simulink model "Juarez_22210417"  (R2023a)
settings: Solver=ode15s  StartTime=0.0  StopTime=30  MaxStep=1e-3  RelTol=1e-3
libraries: slpidlib x1
settings Model: Creator=edang  LastModifiedBy=edang
settings DataIOCC: ReturnWorkspaceOutputs=off  TimeSaveName=t
settings DebuggingCC: AlgebraicLoopMsg=none  ArtificialAlgebraicLoopMsg=none  MaxConsecutiveZCsMsg=none  ModelReferenceExtraNoncontSigs=none  OperatingPointInterfaceChecksumMismatchMsg=none

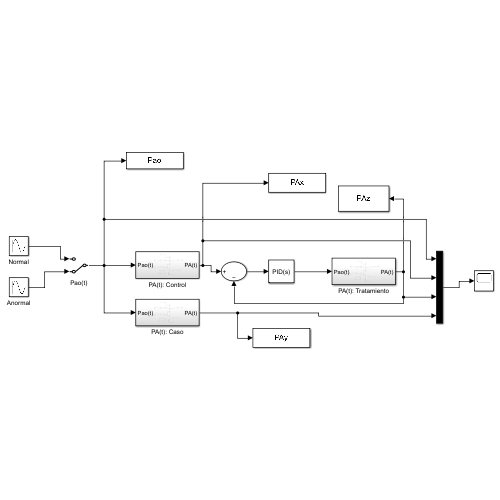
[thumbnail: Simulink's stored preview of the top-level diagram]
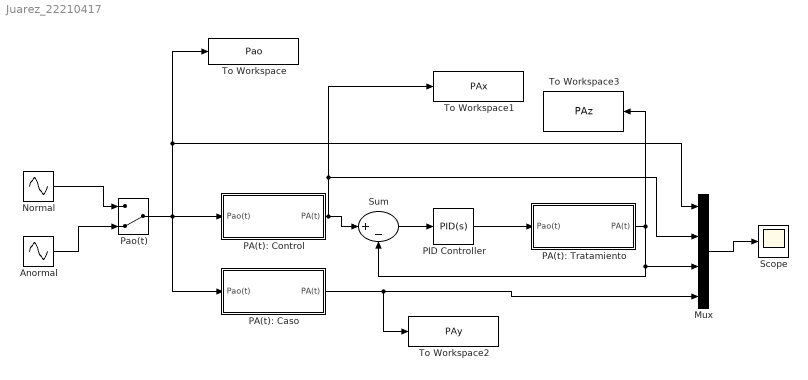
== system Juarez_22210417 ==
  Anormal : Sin  Amplitude=1.5  Frequency=pi/2  SampleTime=0
  Mux : Mux
  Normal : Sin  Amplitude=2.5  Frequency=pi  SampleTime=0
  PA(t): Caso : Subsystem
  PA(t): Control : Subsystem
  PA(t): Tratamiento : Subsystem
  PID Controller : slpidlib/PID Controller  Controller=PID  Form=Parallel  TimeDomain=Continuous-time  UseExternalTs=off  SampleTime=-1  IntegratorMethod=Forward Euler  FilterMethod=Forward Euler  ControllerParametersSource=internal  P=1874.1952  I=62315.7871  UseKiTs=off  D=8.8936  N=202877.133267727  UseFilter=on  TunerSelectOption=Transfer Function Based (PID Tuner App)  InitialConditionSource=internal  InitialConditionForIntegrator=0  InitialConditionForFilter=0  DifferentiatorICPrevScaledInput=0  ExternalReset=none  TrackingMode=off  Kt=1  LimitOutput=off  SatLimitsSource=internal  UpperSaturationLimit=inf  LowerSaturationLimit=-inf  LinearizeAsGain=on  AntiWindupMode=none  Kb=1  LimitIntegrator=off  UpperIntegratorSaturationLimit=inf  LowerIntegratorSaturationLimit=-inf  POutMin=[]  POutMax=[]  IOutMin=[]  IOutMax=[]  DOutMin=[]  DOutMax=[]  NOutMin=[]  NOutMax=[]  SumOutMin=[]  SumOutMax=[]  SaturationOutMin=[]  SaturationOutMax=[]  PParamMin=[]  PParamMax=[]  IParamMin=[]  IParamMax=[]  DParamMin=[]  DParamMax=[]  NParamMin=[]  NParamMax=[]  KbParamMin=[]  KbParamMax=[]  KtParamMin=[]  KtParamMax=[]  KbOutMin=[]  KbOutMax=[]  KtOutMin=[]  KtOutMax=[]  IntegratorOutMin=[]  IntegratorOutMax=[]  FilterOutMin=[]  FilterOutMax=[]  SumI1OutMin=[]  SumI1OutMax=[]  SumI2OutMin=[]  SumI2OutMax=[]  SumI3OutMin=[]  SumI3OutMax=[]  SumI4OutMin=[]  SumI4OutMax=[]  SumDOutMin=[]  SumDOutMax=[]  DifferentiatorOutMin=[]  DifferentiatorOutMax=[]  FilterDiffOutCoefMin=[]  FilterDiffOutCoefMax=[]  ReciprocalOutMin=[]  ReciprocalOutMax=[]  SumDenOutMin=[]  SumDenOutMax=[]  SumNumOutMin=[]  SumNumOutMax=[]  DivideOutMin=[]  DivideOutMax=[]  UdiffTsProdOutMin=[]  UdiffTsProdOutMax=[]  NTsProdOutMin=[]  NTsProdOutMax=[]  UintegralTsProdOutMin=[]  UintegralTsProdOutMax=[]  UngainTsProdOutMin=[]  UngainTsProdOutMax=[]  ClampingZeroOutDataTypeStr=Inherit: Inherit via back propagation  ClampingZeroOutMin=[]  ClampingZeroOutMax=[]  FilterDenConstantOutDataTypeStr=Inherit: Inherit via back propagation  FilterDenConstantOutMin=[]  FilterDenConstantOutMax=[]  PCopyOutDataTypeStr=Inherit: Inherit via back propagation  PCopyOutMin=[]  PCopyOutMax=[]  NCopyOutDataTypeStr=Inherit: Inherit via back propagation  NCopyOutMin=[]  NCopyOutMax=[]  IntegratorContinuousStateAttributes=''  IntegratorStateMustResolveToSignalObject=off  IntegratorRTWStateStorageClass=Auto  FilterContinuousStateAttributes=''  FilterStateMustResolveToSignalObject=off  FilterRTWStateStorageClass=Auto  ParallelPVariant=InternalParameters  IdealPVariant=Disabled  IVariant=InternalParameters  DVariant=InternalParameters  IntegratorVariant=Continuous  SatVariant=Disabled  AWVariant=Passthrough  PCopyVariant=Disabled  TRVariant=Disabled  FdbkBlocksVariant=Forward  IdealPFdbkVariant=Disabled  SatFdbkVariant=Disabled  DerivativeFilterVariant=ContFilter  NVariant=InternalParameters  NCopyVariant=Disabled  FilterICVariant=InternalICsFilter  IntegratorICVariant=InternalICs  ExternalResetVariant=Disabled  TRSumVariant=Passthrough  SumFdbkVariant=Disabled  SumVariant=Sum_PID  TsampFilterVariant=InternalTs  TsampNgainVariant=Passthrough  TsampIntegralVariant=Disabled_SignalSpec  ExternalSaturationOutDataTypeStr=Inherit: Same as second input
  Pao(t) : ManualSwitch  CurrentSetting=0
  Scope : Scope
  Sum : Sum  Inputs=|+-
  To Workspace : ToWorkspace  VariableName=Pao  SampleTime=-1
  To Workspace1 : ToWorkspace  VariableName=PAx  SampleTime=-1
  To Workspace2 : ToWorkspace  VariableName=PAy  SampleTime=-1
  To Workspace3 : ToWorkspace  VariableName=PAz  SampleTime=-1
  wires:
  Normal/1 -> Pao(t)/1
  Anormal/1 -> Pao(t)/2
  Mux/1 -> Scope/1
  Pao(t)/1 -> PA(t): Caso/1(Pao(t)), PA(t): Control/1(Pao(t)), To Workspace/1, Mux/1
  Sum/1 -> PID Controller/1
  PA(t): Control/1(PA(t)) -> To Workspace1/1, Mux/2, Sum/1
  PA(t): Caso/1(PA(t)) -> To Workspace2/1, Mux/4
  PID Controller/1 -> PA(t): Tratamiento/1(Pao(t))
  PA(t): Tratamiento/1(PA(t)) -> Mux/3, Sum/2, To Workspace3/1

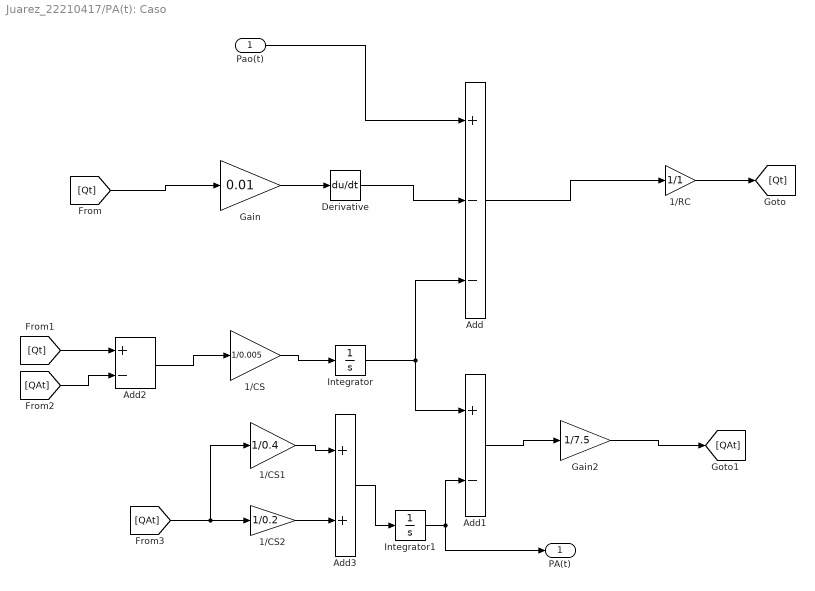
== system Juarez_22210417/PA(t): Caso ==
  Pao(t) : Inport
  1/CS : Gain  Gain=1/0.005
  1/CS1 : Gain  Gain=1/0.4
  1/CS2 : Gain  Gain=1/0.2
  1/RC : Gain  Gain=1/1
  Add : Sum  Inputs=+--
  Add1 : Sum  Inputs=+-
  Add2 : Sum  Inputs=+-
  Add3 : Sum
  Derivative : Derivative
  Gain : Gain  Gain=0.01
  Gain2 : Gain  Gain=1/7.5
  Integrator : Integrator
  Integrator1 : Integrator
  PA(t) : Outport
  wires:
  [QAt] -> 1/CS2/1, 1/CS1/1
  [QAt] -> Add2/2
  Add2/1 -> 1/CS/1
  Add/1 -> 1/RC/1
  Derivative/1 -> Add/2
  1/RC/1 -> [Qt]
  Integrator1/1 -> PA(t)/1, Add1/2
  1/CS1/1 -> Add3/1
  [Qt] -> Gain/1
  Add3/1 -> Integrator1/1
  [Qt] -> Add2/1
  1/CS/1 -> Integrator/1
  Integrator/1 -> Add1/1, Add/3
  1/CS2/1 -> Add3/2
  Add1/1 -> Gain2/1
  Gain/1 -> Derivative/1
  Gain2/1 -> [QAt]
  Pao(t)/1 -> Add/1

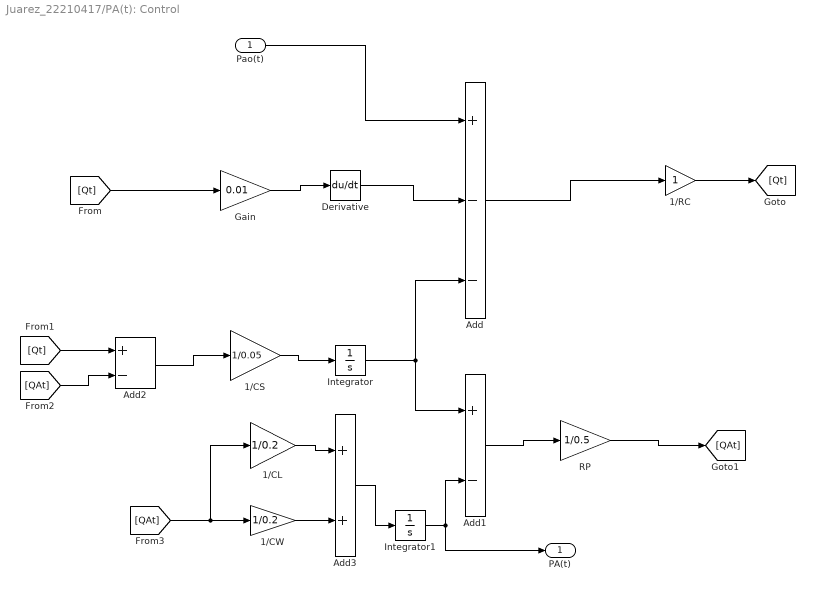
== system Juarez_22210417/PA(t): Control ==
  Pao(t) : Inport
  1/CL : Gain  Gain=1/0.2
  1/CS : Gain  Gain=1/0.05
  1/CW : Gain  Gain=1/0.2
  1/RC : Gain
  Add : Sum  Inputs=+--
  Add1 : Sum  Inputs=+-
  Add2 : Sum  Inputs=+-
  Add3 : Sum
  Derivative : Derivative
  Gain : Gain  Gain=0.01
  Integrator : Integrator
  Integrator1 : Integrator
  RP : Gain  Gain=1/0.5
  PA(t) : Outport
  wires:
  Pao(t)/1 -> Add/1
  Gain/1 -> Derivative/1
  [Qt] -> Gain/1
  Derivative/1 -> Add/2
  Add/1 -> 1/RC/1
  Integrator/1 -> Add1/1, Add/3
  1/CS/1 -> Integrator/1
  Add2/1 -> 1/CS/1
  [Qt] -> Add2/1
  1/RC/1 -> [Qt]
  Add1/1 -> RP/1
  RP/1 -> [QAt]
  1/CL/1 -> Add3/1
  1/CW/1 -> Add3/2
  Add3/1 -> Integrator1/1
  Integrator1/1 -> PA(t)/1, Add1/2
  [QAt] -> 1/CW/1, 1/CL/1
  [QAt] -> Add2/2

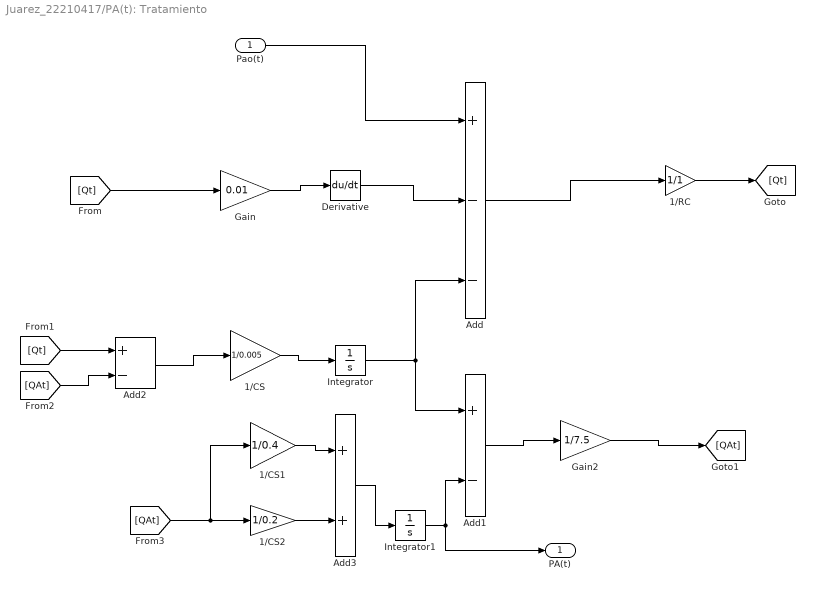
== system Juarez_22210417/PA(t): Tratamiento ==
  Pao(t) : Inport
  1/CS : Gain  Gain=1/0.005
  1/CS1 : Gain  Gain=1/0.4
  1/CS2 : Gain  Gain=1/0.2
  1/RC : Gain  Gain=1/1
  Add : Sum  Inputs=+--
  Add1 : Sum  Inputs=+-
  Add2 : Sum  Inputs=+-
  Add3 : Sum
  Derivative : Derivative
  Gain : Gain  Gain=0.01
  Gain2 : Gain  Gain=1/7.5
  Integrator : Integrator
  Integrator1 : Integrator
  PA(t) : Outport
  wires:
  [QAt] -> 1/CS2/1, 1/CS1/1
  [QAt] -> Add2/2
  Add2/1 -> 1/CS/1
  Add/1 -> 1/RC/1
  Derivative/1 -> Add/2
  1/RC/1 -> [Qt]
  Integrator1/1 -> PA(t)/1, Add1/2
  1/CS1/1 -> Add3/1
  [Qt] -> Gain/1
  Add3/1 -> Integrator1/1
  [Qt] -> Add2/1
  1/CS/1 -> Integrator/1
  Integrator/1 -> Add1/1, Add/3
  1/CS2/1 -> Add3/2
  Add1/1 -> Gain2/1
  Gain/1 -> Derivative/1
  Gain2/1 -> [QAt]
  Pao(t)/1 -> Add/1
